simulink model "open_loop_motor"  (R2022b)
settings: Solver=FixedStepDiscrete  StartTime=0.0  StopTime=60  FixedStep=10e-3  MaxStep=5e-3  RelTol=1e-3  EnableMultiTasking=on
libraries: arduinolib x3, arduinosensorlib x1
settings Model: ExtModeTrigDuration=2  Creator=ZMS  LastModifiedBy=ZMS
settings OptimizationCC: EnhancedBackFolding=on  PassReuseOutputArgsAs=Individual arguments  ZeroExternalMemoryAtStartup=off  ZeroInternalMemoryAtStartup=off  MaxStackSize=64  OptimizeBlockOrder=speed  DifferentSizesBufferReuse=on  OptimizationCustomize=off  EfficientTunableParamExpr=on
settings DebuggingCC: ParameterTunabilityLossMsg=error
settings HardwareCC: ProdBitPerInt=16  ProdBitPerPointer=16  ProdBitPerSizeT=16  ProdBitPerPtrDiffT=16  ProdLargestAtomicFloat=None  ProdWordSize=8  ProdHWDeviceType=Atmel->AVR  UseEmbeddedCoderFeatures=off  UseSimulinkCoderFeatures=off
settings SFSimCC: MATLABDynamicMemAlloc=off
settings RTWCC: Description=Embedded Coder  SystemTargetFile=ert.tlc  HardwareBoard=Arduino Mega 2560  TLCOptions="-aInlineSetEventsForThisBaseRateFcn=TLC_FALSE -aSuppressMultiTaskScheduler=TLC_FALSE     -aRateBasedStepFcn=1"  TemplateMakefile=ert_default_tmf  Toolchain=Arduino AVR  BuildConfiguration=Faster Runs
settings CodeAppCC: ForceParamTrailComments=on  IgnoreCustomStorageClasses=off  OperatorAnnotations=on  SimulinkDataObjDesc=on  SFDataObjDesc=on  InsertBlockDesc=on
settings ERTTargetCC: SupportContinuousTime=on  SupportNonInlinedSFcns=on  SupportVariableSizeSignals=on  ExtModeTransport=3  ExtModeStaticAlloc=on  ExtModeAutomaticAllocSize=off  ExtModeStaticAllocSize=2048  ExtModeMexFile=ext_xcp  ExtModeIntrfLevel=Level2 - Open

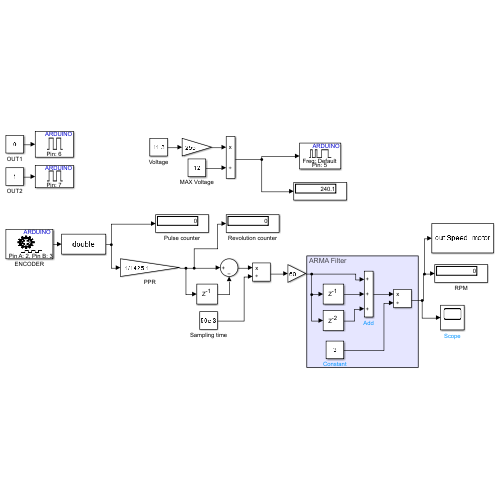
[thumbnail: Simulink's stored preview of the top-level diagram]
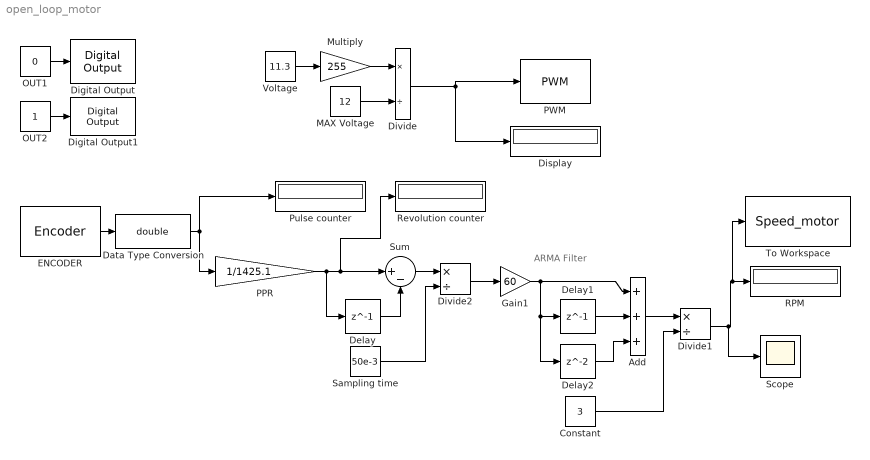
== system open_loop_motor ==
  note: ARMA Filter
  Add : Sum  Inputs=+++
  Constant : Constant  Value=3
  Data Type Conversion : DataTypeConversion  OutDataTypeStr=double  SaturateOnIntegerOverflow=off  RndMeth=Floor
  Delay : Delay  DelayLength=1
  Delay1 : Delay  DelayLength=1
  Delay2 : Delay
  Digital Output : arduinolib/Digital Output  pinNumber=6  Direction=output  blockPlatform=arduino
  Digital Output1 : arduinolib/Digital Output  pinNumber=7  Direction=output  blockPlatform=arduino
  Display : Display
  Divide : Product  Inputs=*/
  Divide1 : Product  Inputs=*/
  Divide2 : Product  Inputs=*/
  ENCODER : arduinosensorlib/Encoder  InputA=2  InputB=3  Mode=No reset  SampleTime=-1
  Gain1 : Gain  Gain=60
  MAX Voltage : Constant  Value=12
  Multiply : Gain  Gain=255
  OUT1 : Constant  Value=0
  OUT2 : Constant
  PPR : Gain  Gain=1/1425.1
  PWM : arduinolib/PWM  pinNumber=5  frequencyType=Default  desiredFrequency=50  achievableFrequency=50
  Pulse counter : Display
  RPM : Display
  Revolution counter : Display
  Sampling time : Constant  Value=50e-3
  Scope : Scope
  Sum : Sum  Inputs=|+-
  To Workspace : ToWorkspace  VariableName=Speed_motor  SampleTime=-1
      settings: Save2DSignal=2-D array (concatenate along first dimension)
  Voltage : Constant  Value=11.3
  wires:
  Voltage/1 -> Multiply/1
  Multiply/1 -> Divide/1
  Divide/1 -> Display/1, PWM/1
  MAX Voltage/1 -> Divide/2
  ENCODER/1 -> Data Type Conversion/1
  Data Type Conversion/1 -> Pulse counter/1, PPR/1
  PPR/1 -> Sum/1, Revolution counter/1, Delay/1
  Sum/1 -> Divide2/1
  Divide2/1 -> Gain1/1
  Sampling time/1 -> Divide2/2
  Delay/1 -> Sum/2
  OUT1/1 -> Digital Output/1
  OUT2/1 -> Digital Output1/1
  Gain1/1 -> Delay1/1, Delay2/1, Add/1
  Delay1/1 -> Add/2
  Delay2/1 -> Add/3
  Add/1 -> Divide1/1
  Divide1/1 -> Scope/1, To Workspace/1, RPM/1
  Constant/1 -> Divide1/2
